simulink model "exp5_5"  (Simulink 3.00)
settings: Solver=ode45  SolverMode=SingleTasking  StartTime=0.0  StopTime=10.0  RelTol=1e-3  AbsTol=1e-6
settings Model: RTWTemplateMakefile=grt_vc.tmf

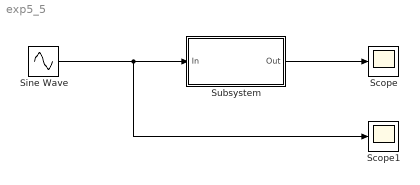
== system exp5_5 ==
  Scope : Scope
      settings: TickLabels=on  TimeRange=10  YMin=-5  YMax=10  SaveToWorkspace=off  SaveName=ScopeData  DataFormat=Matrix
  Scope1 : Scope
      settings: TickLabels=on  TimeRange=10  YMin=-1  YMax=1  SaveToWorkspace=off  SaveName=ScopeData  DataFormat=Matrix
  Sine Wave : Sin  Amplitude=1  Frequency=1  Phase=0  SampleTime=0
  Subsystem : Subsystem
  wires:
  Sine Wave/1 -> Subsystem/1(In), Scope1/1
  Subsystem/1(Out) -> Scope/1

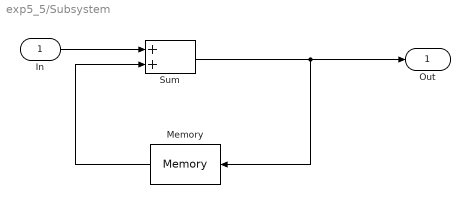
== system exp5_5/Subsystem ==
  In : Inport  Port=1  PortWidth=-1  SampleTime=-1  DataType=auto
      settings: SignalType=auto
  Memory : Memory  Orientation=left  X0=0  InheritSampleTime=off
  Sum : Sum  Inputs=++  SaturateOnIntegerOverflow=on
  Out : Outport  Port=1  InitialOutput=0
  wires:
  Memory/1 -> Sum/2
  Sum/1 -> Memory/1, Out/1
  In/1 -> Sum/1
